simulink model "induction_motor"  (Simulink 5.0)
settings: Solver=ode45  StartTime=0.0  StopTime=1  RelTol=1e-3
libraries: simulink x1
settings Model: LastModifiedBy=JBB

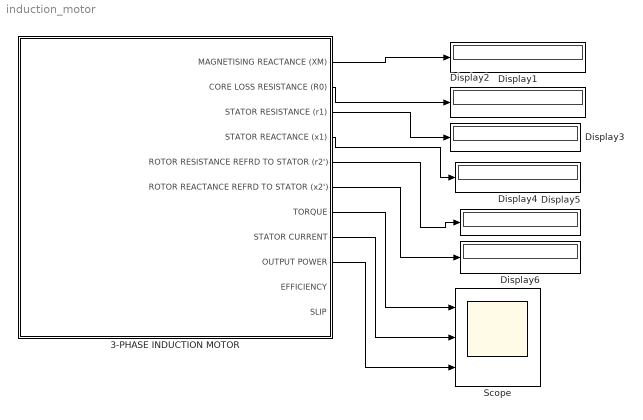
== system induction_motor ==
  3-PHASE INDUCTION MOTOR : Subsystem  mask(Squirrel cage Induction motor){w=3*746, v=415, f=50, P=4, c=DELTA, m=CLASS A, I_NL=3.04, V_NL=415, P_NL=232, I_BR=5, V_BR=84, P_BR=433, r1=7.5}
      mask prompts: w "Nominal Power ( w)"; v "Rated voltage (Volt)"; f "Frequency (Hz)"; P "No. Of poles"; c "Stator connection"; m "Class of Motor"; I_NL "No Load Line current (Amp)"; V_NL "No Load Line Voltage (Volt)"; P_NL "No Load Power (Watt)"; I_BR "Blocked Rotor Line Current (Amp)"; V_BR "Blocked Rotor  Line Voltage (Volt)"; P_BR "Blocked Rotor Power (Watt)"; r1 "Stator Resistance (From DC Test)"
      mask help:
      | Implements a three-phase asynchronous machine ( squirrel cage).
      | The motor test results (No Load, Blocked rotor & DC stator resistance test) are used to get the performance characteristics of the motor.
      mask init:
      | switch c
      | case 1
      |     s = 3;
      |     d = 1;
      | case 2
      |     s=1;
      |     d=3;
      | end
      | switch m
      | case 1
      | 	m=0.5;
      | case 2
      | 	m=0.4;
      | case 3
      | 	m=0.3
      | case 4
      | 	m=0.5
      | end
      mask StyleString: edit,edit,edit,edit,popup(STAR|DELTA),popup(CLASS A|CLASS B|CLASS C|CLASS D),edit,edit,edit,edit,edit,edit,edit
  Display{1..6} (6 alike) : Display
  Scope : Scope  NumInputPorts=3
      settings: TimeRange=1  YMin=-6~-5~-5  YMax=12~5~5
  wires:
  3-PHASE INDUCTION MOTOR/1(MAGNETISING REACTANCE (XM)) -> Display1/1
  3-PHASE INDUCTION MOTOR/2(CORE LOSS RESISTANCE (R0)) -> Display2/1
  3-PHASE INDUCTION MOTOR/3(STATOR RESISTANCE (r1)) -> Display3/1
  3-PHASE INDUCTION MOTOR/4(STATOR REACTANCE (x1)) -> Display4/1
  3-PHASE INDUCTION MOTOR/5(ROTOR RESISTANCE REFRD TO STATOR (r2')) -> Display5/1
  3-PHASE INDUCTION MOTOR/6(ROTOR REACTANCE REFRD TO STATOR (x2')) -> Display6/1
  3-PHASE INDUCTION MOTOR/7(TORQUE) -> Scope/1
  3-PHASE INDUCTION MOTOR/8(STATOR CURRENT) -> Scope/2
  3-PHASE INDUCTION MOTOR/9(OUTPUT POWER) -> Scope/3

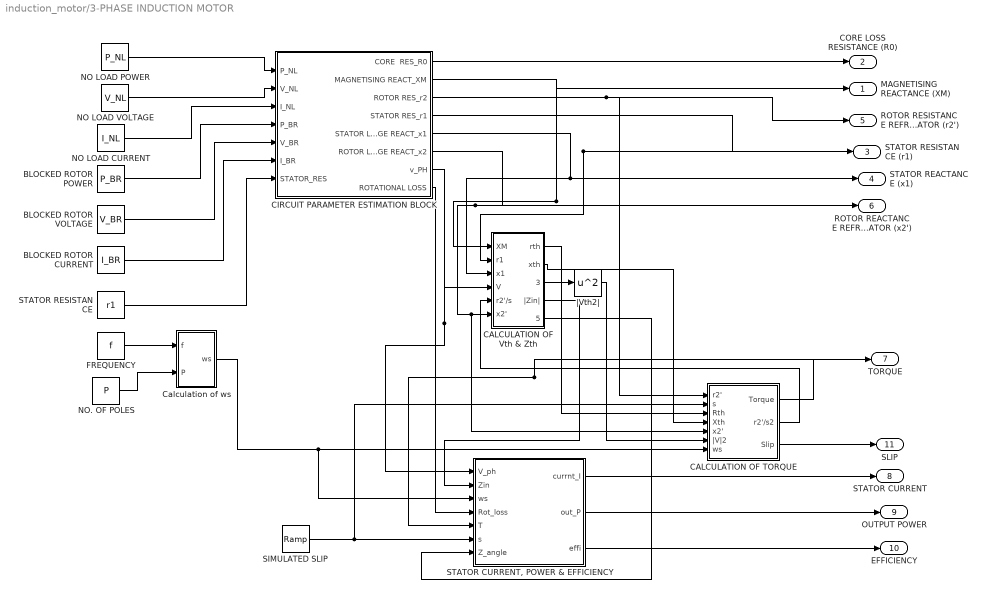
== system induction_motor/3-PHASE INDUCTION MOTOR ==
  BLOCKED ROTOR CURRENT : Constant  Value=I_BR
  BLOCKED ROTOR POWER : Constant  Value=P_BR
  BLOCKED ROTOR VOLTAGE : Constant  Value=V_BR
  CALCULATION OF TORQUE : Subsystem
  CALCULATION OF Vth & Zth : Subsystem
  CIRCUIT PARAMETER ESTIMATION BLOCK : Subsystem
  Calculation of ws : Subsystem
  FREQUENCY : Constant  Value=f
  NO LOAD CURRENT : Constant  Value=I_NL
  NO LOAD POWER : Constant  Value=P_NL
  NO LOAD VOLTAGE : Constant  Value=V_NL
  NO. OF POLES : Constant  Value=P
  SIMULATED SLIP : simulink/Sources/Ramp  slope=1  start=0  X0=0.001
  "STATOR CURRENT, POWER & EFFICIENCY" : Subsystem
  STATOR RESISTANCE : Constant  Value=r1
  |Vth2| : Math  Operator=square
  MAGNETISING REACTANCE (XM) : Outport
  CORE LOSS RESISTANCE (R0) : Outport  Port=2
  STATOR RESISTANCE (r1) : Outport  Port=3
  STATOR REACTANCE (x1) : Outport  Port=4
  ROTOR RESISTANCE REFRD TO STATOR (r2') : Outport  Port=5
  ROTOR REACTANCE REFRD TO STATOR (x2') : Outport  Port=6
  TORQUE : Outport  Port=7
  STATOR CURRENT : Outport  Port=8
  OUTPUT POWER : Outport  Port=9
  EFFICIENCY : Outport  Port=10
  SLIP : Outport  Port=11
  wires:
  CIRCUIT PARAMETER ESTIMATION BLOCK/1(CORE  RES_R0) -> CORE LOSS RESISTANCE (R0)/1
  CIRCUIT PARAMETER ESTIMATION BLOCK/2(MAGNETISING REACT_XM) -> MAGNETISING REACTANCE (XM)/1, CALCULATION OF Vth & Zth/1(XM)
  CIRCUIT PARAMETER ESTIMATION BLOCK/3(ROTOR RES_r2) -> CALCULATION OF TORQUE/1(r2'), ROTOR RESISTANCE REFRD TO STATOR (r2')/1
  CIRCUIT PARAMETER ESTIMATION BLOCK/4(STATOR RES_r1) -> CALCULATION OF Vth & Zth/2(r1), STATOR RESISTANCE (r1)/1
  CIRCUIT PARAMETER ESTIMATION BLOCK/5(STATOR LEAKAGE REACT_x1) -> STATOR REACTANCE (x1)/1, CALCULATION OF Vth & Zth/3(x1)
  CIRCUIT PARAMETER ESTIMATION BLOCK/6(ROTOR LEAKAGE REACT_x2) -> ROTOR REACTANCE REFRD TO STATOR (x2')/1, CALCULATION OF TORQUE/5(x2'), CALCULATION OF Vth & Zth/6(x2')
  NO LOAD CURRENT/1 -> CIRCUIT PARAMETER ESTIMATION BLOCK/3(I_NL)
  NO LOAD POWER/1 -> CIRCUIT PARAMETER ESTIMATION BLOCK/1(P_NL)
  BLOCKED ROTOR CURRENT/1 -> CIRCUIT PARAMETER ESTIMATION BLOCK/6(I_BR)
  BLOCKED ROTOR POWER/1 -> CIRCUIT PARAMETER ESTIMATION BLOCK/4(P_BR)
  BLOCKED ROTOR VOLTAGE/1 -> CIRCUIT PARAMETER ESTIMATION BLOCK/5(V_BR)
  NO. OF POLES/1 -> Calculation of ws/2(P)
  STATOR RESISTANCE/1 -> CIRCUIT PARAMETER ESTIMATION BLOCK/7(STATOR_RES)
  CALCULATION OF Vth & Zth/3(|VTH|) -> |Vth2|/1
  SIMULATED SLIP/1 -> CALCULATION OF TORQUE/2(s), "STATOR CURRENT, POWER & EFFICIENCY"/6(s)
  CALCULATION OF Vth & Zth/1(rth) -> CALCULATION OF TORQUE/3(Rth)
  CALCULATION OF Vth & Zth/2(xth) -> CALCULATION OF TORQUE/4(Xth)
  |Vth2|/1 -> CALCULATION OF TORQUE/6(|V|2)
  Calculation of ws/1(ws) -> CALCULATION OF TORQUE/7(ws), "STATOR CURRENT, POWER & EFFICIENCY"/3(ws)
  CALCULATION OF TORQUE/1(Torque) -> TORQUE/1, "STATOR CURRENT, POWER & EFFICIENCY"/5(T)
  CALCULATION OF TORQUE/2(r2'/s2) -> CALCULATION OF Vth & Zth/5(r2'/s)
  CALCULATION OF Vth & Zth/4(|Zin|) -> "STATOR CURRENT, POWER & EFFICIENCY"/2(Zin)
  "STATOR CURRENT, POWER & EFFICIENCY"/3(effi) -> EFFICIENCY/1
  "STATOR CURRENT, POWER & EFFICIENCY"/1(currnt_I) -> STATOR CURRENT/1
  "STATOR CURRENT, POWER & EFFICIENCY"/2(out_P) -> OUTPUT POWER/1
  CIRCUIT PARAMETER ESTIMATION BLOCK/7(v_PH) -> CALCULATION OF Vth & Zth/4(V), "STATOR CURRENT, POWER & EFFICIENCY"/1(V_ph)
  CALCULATION OF Vth & Zth/5(Z_angle) -> "STATOR CURRENT, POWER & EFFICIENCY"/7(Z_angle)
  CALCULATION OF TORQUE/3(Slip) -> SLIP/1
  NO LOAD VOLTAGE/1 -> CIRCUIT PARAMETER ESTIMATION BLOCK/2(V_NL)
  FREQUENCY/1 -> Calculation of ws/1(f)
  CIRCUIT PARAMETER ESTIMATION BLOCK/8(ROTATIONAL LOSS) -> "STATOR CURRENT, POWER & EFFICIENCY"/4(Rot_loss)

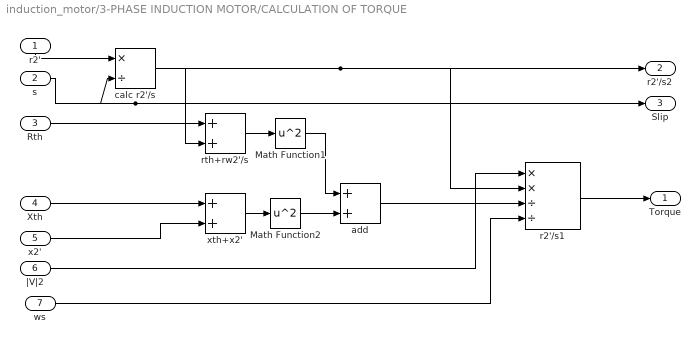
== system induction_motor/3-PHASE INDUCTION MOTOR/CALCULATION OF TORQUE ==
  r2' : Inport  Orientation=down
  s : Inport  Port=2
  Rth : Inport  Port=3
  Xth : Inport  Port=4
  x2' : Inport  Port=5
  |V|2 : Inport  Port=6
  ws : Inport  Port=7
  Math Function1 : Math  Operator=square
  Math Function2 : Math  Operator=square
  add : Sum  ShowAdditionalParam=on  OutDataTypeMode=double  OutScaling=2^-10
  calc r2'/s : Product  Inputs=*/  ShowAdditionalParam=on  OutDataTypeMode=double  OutScaling=2^-10
  r2'/s1 : Product  Inputs=**//  ShowAdditionalParam=on  OutDataTypeMode=double  OutScaling=2^-10
  rth+rw2'/s : Sum  ShowAdditionalParam=on  OutDataTypeMode=double  OutScaling=2^-10
  xth+x2' : Sum  ShowAdditionalParam=on  OutDataTypeMode=double  OutScaling=2^-10
  Torque : Outport
  r2'/s2 : Outport  Port=2
  Slip : Outport  Port=3
  wires:
  calc r2'/s/1 -> rth+rw2'/s/2, r2'/s1/2, r2'/s2/1
  rth+rw2'/s/1 -> Math Function1/1
  xth+x2'/1 -> Math Function2/1
  Math Function1/1 -> add/1
  Math Function2/1 -> add/2
  add/1 -> r2'/s1/3
  r2'/1 -> calc r2'/s/1
  x2'/1 -> xth+x2'/2
  s/1 -> calc r2'/s/2, Slip/1
  Rth/1 -> rth+rw2'/s/1
  Xth/1 -> xth+x2'/1
  |V|2/1 -> r2'/s1/1
  r2'/s1/1 -> Torque/1
  ws/1 -> r2'/s1/4

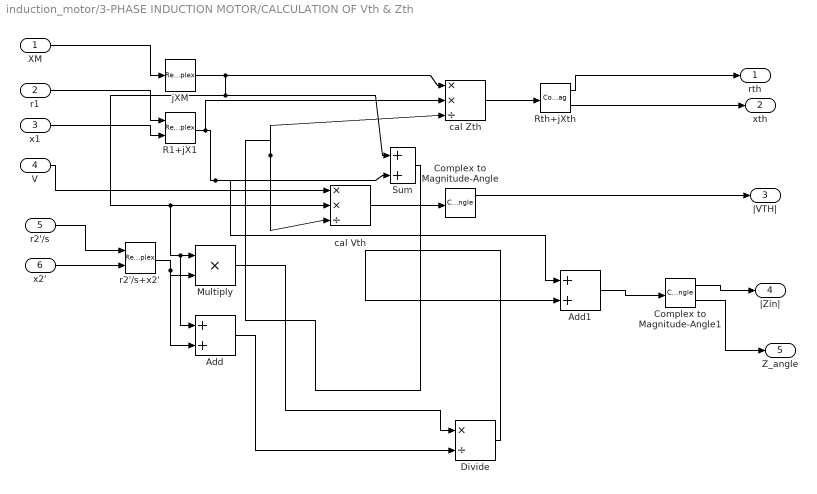
== system induction_motor/3-PHASE INDUCTION MOTOR/CALCULATION OF Vth & Zth ==
  XM : Inport
  r1 : Inport  Port=2
  x1 : Inport  Port=3
  V : Inport  Port=4
  r2'/s : Inport  Port=5
  x2' : Inport  Port=6
  Add : Sum  ShowAdditionalParam=on  OutDataTypeMode=double  OutScaling=2^-10
  Add1 : Sum  ShowAdditionalParam=on  OutDataTypeMode=double  OutScaling=2^-10
  Complex to Magnitude-Angle : ComplexToMagnitudeAngle
  Complex to Magnitude-Angle1 : ComplexToMagnitudeAngle
  Divide : Product  Inputs=*/  ShowAdditionalParam=on  OutDataTypeMode=double  OutScaling=2^-10
  Multiply : Product  Inputs=**  ShowAdditionalParam=on  OutDataTypeMode=double  OutScaling=2^-10
  R1+jX1 : RealImagToComplex
  Rth+jXth : ComplexToRealImag
  Sum : Sum  Inputs=|++  SaturateOnIntegerOverflow=on
  cal Vth : Product  Inputs=**/  ShowAdditionalParam=on  OutDataTypeMode=double  OutDataType=float('single')  OutScaling=2^-10
  cal Zth : Product  Inputs=**/  ShowAdditionalParam=on  OutDataType=float('single')  OutScaling=2^-10
  jXM : RealImagToComplex  Input=Imag
  r2'/s+x2' : RealImagToComplex
  rth : Outport
  xth : Outport  Port=2
  |VTH| : Outport  Port=3
  |Zin| : Outport  Port=4
  Z_angle : Outport  Port=5
  wires:
  jXM/1 -> cal Zth/1, Sum/1, cal Vth/2, Multiply/1, Add/1
  R1+jX1/1 -> cal Zth/2, Add1/1, Sum/2
  Sum/1 -> cal Zth/3, cal Vth/3
  XM/1 -> jXM/1
  r1/1 -> R1+jX1/1
  x1/1 -> R1+jX1/2
  V/1 -> cal Vth/1
  cal Zth/1 -> Rth+jXth/1
  Rth+jXth/1 -> rth/1
  Rth+jXth/2 -> xth/1
  cal Vth/1 -> Complex to Magnitude-Angle/1
  Complex to Magnitude-Angle/1 -> |VTH|/1
  r2'/s/1 -> r2'/s+x2'/1
  x2'/1 -> r2'/s+x2'/2
  r2'/s+x2'/1 -> Multiply/2, Add/2
  Multiply/1 -> Divide/1
  Add/1 -> Divide/2
  Divide/1 -> Add1/2
  Add1/1 -> Complex to Magnitude-Angle1/1
  Complex to Magnitude-Angle1/1 -> |Zin|/1
  Complex to Magnitude-Angle1/2 -> Z_angle/1

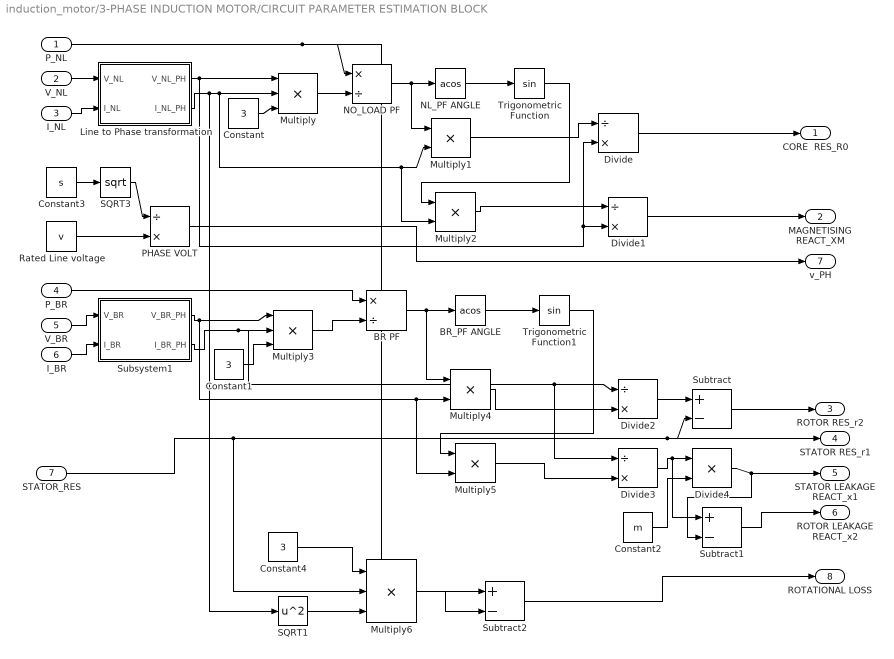
== system induction_motor/3-PHASE INDUCTION MOTOR/CIRCUIT PARAMETER ESTIMATION BLOCK ==
  P_NL : Inport
  V_NL : Inport  Port=2
  I_NL : Inport  Port=3
  P_BR : Inport  Port=4
  V_BR : Inport  Port=5
  I_BR : Inport  Port=6
  STATOR_RES : Inport  Port=7
  BR PF : Product  Inputs=*/  ShowAdditionalParam=on  OutDataTypeMode=Specify via dialog  OutDataType=float('single')  OutScaling=2^-10
  BR_PF ANGLE : Trigonometry  Operator=acos
  Constant : Constant  Value=3
  Constant1 : Constant  Value=3
  Constant2 : Constant  Value=m
  Constant3 : Constant  Value=s
  Constant4 : Constant  Value=3
  Divide : Product  Inputs=/*  ShowAdditionalParam=on  OutDataTypeMode=double  OutDataType=float('single')  OutScaling=2^-10
  Divide1 : Product  Inputs=/*  ShowAdditionalParam=on  OutDataTypeMode=double  OutDataType=float('single')  OutScaling=2^-10
  Divide2 : Product  Inputs=/*  ShowAdditionalParam=on  OutDataTypeMode=Specify via dialog  OutDataType=float('single')  OutScaling=2^-10
  Divide3 : Product  Inputs=/*  ShowAdditionalParam=on  OutDataTypeMode=Specify via dialog  OutDataType=float('single')  OutScaling=2^-10
  Divide4 : Product  Inputs=**  ShowAdditionalParam=on  OutDataTypeMode=double  OutDataType=float('single')  OutScaling=2^-10
  Line to Phase transformation : Subsystem
  Multiply : Product  Inputs=***  ShowAdditionalParam=on  OutDataTypeMode=double  OutDataType=float('single')  OutScaling=2^-10
  Multiply{1..2,4..5} (4 alike) : Product  Inputs=**  ShowAdditionalParam=on  OutDataTypeMode=Specify via dialog  OutDataType=float('single')  OutScaling=2^-10
  Multiply3 : Product  Inputs=***  ShowAdditionalParam=on  OutDataTypeMode=double  OutDataType=float('single')  OutScaling=2^-10
  Multiply6 : Product  Inputs=***  ShowAdditionalParam=on  OutDataTypeMode=Specify via dialog  OutDataType=float('single')  OutScaling=2^-10
  NL_PF ANGLE : Trigonometry  Operator=acos
  NO_LOAD PF : Product  Inputs=*/  ShowAdditionalParam=on  OutDataTypeMode=Specify via dialog  OutDataType=float('single')  OutScaling=2^-10
  PHASE VOLT : Product  Inputs=/*  ShowAdditionalParam=on  OutDataTypeMode=double  OutDataType=float('single')  OutScaling=2^-10
  Rated Line voltage : Constant  Value=v
  SQRT1 : Math  Operator=square
  SQRT3 : Math  Operator=sqrt
  Subsystem1 : Subsystem
  Subtract : Sum  Inputs=+-  ShowAdditionalParam=on  OutDataTypeMode=double  OutDataType=float('single')  OutScaling=2^-10
  Subtract1 : Sum  Inputs=+-  ShowAdditionalParam=on  OutDataTypeMode=double  OutDataType=float('single')  OutScaling=2^-10
  Subtract2 : Sum  Inputs=+-  ShowAdditionalParam=on  OutDataTypeMode=Specify via dialog  OutDataType=float('single')  OutScaling=2^-10
  Trigonometric Function : Trigonometry
  Trigonometric Function1 : Trigonometry
  CORE  RES_R0 : Outport
  MAGNETISING REACT_XM : Outport  Port=2
  ROTOR RES_r2 : Outport  Port=3
  STATOR RES_r1 : Outport  Port=4
  STATOR LEAKAGE REACT_x1 : Outport  Port=5
  ROTOR LEAKAGE REACT_x2 : Outport  Port=6
  v_PH : Outport  Port=7
  ROTATIONAL LOSS : Outport  Port=8
  wires:
  P_NL/1 -> NO_LOAD PF/1, Subtract2/1
  Multiply/1 -> NO_LOAD PF/2
  NO_LOAD PF/1 -> NL_PF ANGLE/1, Multiply1/1
  Divide/1 -> CORE  RES_R0/1
  Multiply2/1 -> Divide1/1
  NL_PF ANGLE/1 -> Trigonometric Function/1
  Divide1/1 -> MAGNETISING REACT_XM/1
  P_BR/1 -> BR PF/1
  BR_PF ANGLE/1 -> Trigonometric Function1/1
  Divide2/1 -> Subtract/1
  Subtract/1 -> ROTOR RES_r2/1
  Divide4/1 -> STATOR LEAKAGE REACT_x1/1, Subtract1/2
  I_NL/1 -> Line to Phase transformation/2(I_NL)
  V_NL/1 -> Line to Phase transformation/1(V_NL)
  Line to Phase transformation/1(V_NL_PH) -> Multiply/1, Divide/2, Divide1/2
  Line to Phase transformation/2(I_NL_PH) -> Multiply/2, Multiply1/2, Multiply2/2, SQRT1/1
  Constant/1 -> Multiply/3
  Trigonometric Function/1 -> Multiply2/1
  Multiply1/1 -> Divide/1
  V_BR/1 -> Subsystem1/1(V_BR)
  I_BR/1 -> Subsystem1/2(I_BR)
  Subsystem1/1(V_BR_PH) -> Multiply4/2, Multiply5/2, Multiply3/1
  Subsystem1/2(I_BR_PH) -> Multiply3/2, Divide2/1, Divide3/1
  Constant1/1 -> Multiply3/3
  Multiply3/1 -> BR PF/2
  BR PF/1 -> BR_PF ANGLE/1, Multiply4/1
  Trigonometric Function1/1 -> Multiply5/1
  Divide3/1 -> Divide4/1, Subtract1/1
  Constant2/1 -> Divide4/2
  STATOR_RES/1 -> Subtract/2, STATOR RES_r1/1, Multiply6/2
  Constant3/1 -> SQRT3/1
  SQRT3/1 -> PHASE VOLT/1
  Rated Line voltage/1 -> PHASE VOLT/2
  PHASE VOLT/1 -> v_PH/1
  Subtract1/1 -> ROTOR LEAKAGE REACT_x2/1
  Constant4/1 -> Multiply6/1
  Multiply6/1 -> Subtract2/2
  SQRT1/1 -> Multiply6/3
  Subtract2/1 -> ROTATIONAL LOSS/1
  Multiply4/1 -> Divide2/2
  Multiply5/1 -> Divide3/2

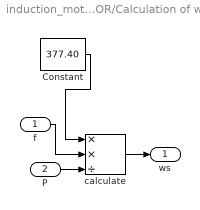
== system induction_motor/3-PHASE INDUCTION MOTOR/Calculation of ws ==
  f : Inport
  P : Inport  Port=2
  Constant : Constant  Value=377.40
  calculate : Product  Inputs=**/  ShowAdditionalParam=on  OutDataTypeMode=double  OutDataType=float('single')  OutScaling=2^-10
  ws : Outport
  wires:
  Constant/1 -> calculate/1
  f/1 -> calculate/2
  calculate/1 -> ws/1
  P/1 -> calculate/3

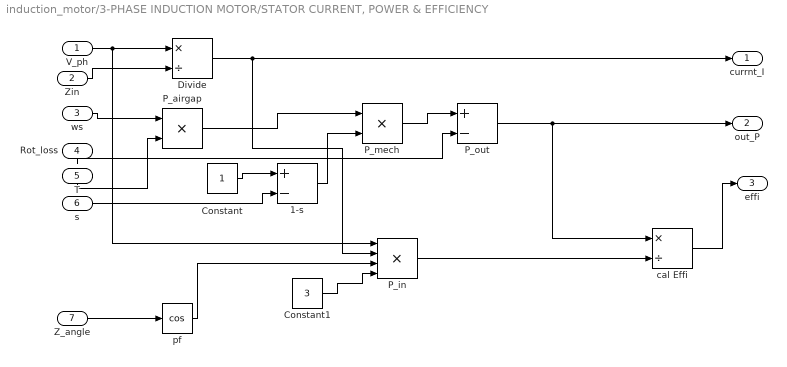
== system induction_motor/3-PHASE INDUCTION MOTOR/STATOR CURRENT, POWER & EFFICIENCY ==
  V_ph : Inport
  Zin : Inport  Port=2
  ws : Inport  Port=3
  Rot_loss : Inport  Orientation=down  Port=4
  T : Inport  Orientation=down  Port=5
  s : Inport  Port=6
  Z_angle : Inport  Port=7
  1-s : Sum  Inputs=+-  ShowAdditionalParam=on  OutDataTypeMode=double  OutScaling=2^-10
  Constant : Constant
  Constant1 : Constant  Value=3
  Divide : Product  Inputs=*/  ShowAdditionalParam=on  OutDataTypeMode=double  OutScaling=2^-10
  P_airgap : Product  Inputs=**  ShowAdditionalParam=on  OutDataTypeMode=double  OutScaling=2^-10
  P_in : Product  Inputs=****  ShowAdditionalParam=on  OutDataTypeMode=double  OutScaling=2^-10
  P_mech : Product  Inputs=**  ShowAdditionalParam=on  OutDataTypeMode=double  OutScaling=2^-10
  P_out : Sum  Inputs=+-  ShowAdditionalParam=on  OutDataTypeMode=double  OutScaling=2^-10
  cal Effi : Product  Inputs=*/  ShowAdditionalParam=on  OutDataTypeMode=double  OutScaling=2^-10
  pf : Trigonometry  Operator=cos
  currnt_I : Outport
  out_P : Outport  Port=2
  effi : Outport  Port=3
  wires:
  Divide/1 -> P_in/2, currnt_I/1
  Constant/1 -> 1-s/1
  P_airgap/1 -> P_mech/1
  1-s/1 -> P_mech/2
  P_mech/1 -> P_out/1
  Constant1/1 -> P_in/4
  pf/1 -> P_in/3
  P_out/1 -> cal Effi/1, out_P/1
  P_in/1 -> cal Effi/2
  V_ph/1 -> Divide/1, P_in/1
  ws/1 -> P_airgap/1
  Rot_loss/1 -> P_out/2
  T/1 -> P_airgap/2
  s/1 -> 1-s/2
  Zin/1 -> Divide/2
  cal Effi/1 -> effi/1
  Z_angle/1 -> pf/1

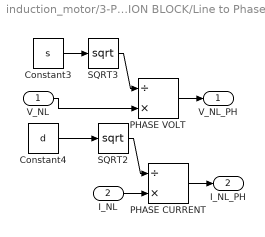
== system induction_motor/3-PHASE INDUCTION MOTOR/CIRCUIT PARAMETER ESTIMATION BLOCK/Line to Phase transformation ==
  V_NL : Inport
  I_NL : Inport  Port=2
  Constant3 : Constant  Value=s
  Constant4 : Constant  Value=d
  PHASE CURRENT : Product  Inputs=/*  ShowAdditionalParam=on  OutDataTypeMode=double  OutDataType=float('single')  OutScaling=2^-10
  PHASE VOLT : Product  Inputs=/*  ShowAdditionalParam=on  OutDataTypeMode=double  OutDataType=float('single')  OutScaling=2^-10
  SQRT2 : Math  Operator=sqrt
  SQRT3 : Math  Operator=sqrt
  V_NL_PH : Outport
  I_NL_PH : Outport  Port=2
  wires:
  Constant3/1 -> SQRT3/1
  SQRT3/1 -> PHASE VOLT/1
  Constant4/1 -> SQRT2/1
  SQRT2/1 -> PHASE CURRENT/1
  PHASE VOLT/1 -> V_NL_PH/1
  V_NL/1 -> PHASE VOLT/2
  PHASE CURRENT/1 -> I_NL_PH/1
  I_NL/1 -> PHASE CURRENT/2

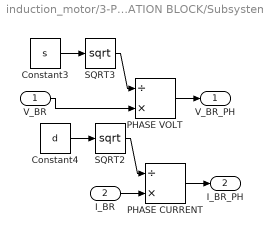
== system induction_motor/3-PHASE INDUCTION MOTOR/CIRCUIT PARAMETER ESTIMATION BLOCK/Subsystem1 ==
  V_BR : Inport
  I_BR : Inport  Port=2
  Constant3 : Constant  Value=s
  Constant4 : Constant  Value=d
  PHASE CURRENT : Product  Inputs=/*  ShowAdditionalParam=on  OutDataTypeMode=double  OutDataType=float('single')  OutScaling=2^-10
  PHASE VOLT : Product  Inputs=/*  ShowAdditionalParam=on  OutDataTypeMode=double  OutDataType=float('single')  OutScaling=2^-10
  SQRT2 : Math  Operator=sqrt
  SQRT3 : Math  Operator=sqrt
  V_BR_PH : Outport
  I_BR_PH : Outport  Port=2
  wires:
  Constant3/1 -> SQRT3/1
  SQRT3/1 -> PHASE VOLT/1
  Constant4/1 -> SQRT2/1
  SQRT2/1 -> PHASE CURRENT/1
  PHASE VOLT/1 -> V_BR_PH/1
  V_BR/1 -> PHASE VOLT/2
  PHASE CURRENT/1 -> I_BR_PH/1
  I_BR/1 -> PHASE CURRENT/2
